simulink model "TST_ECBtn_DD"  (R2016b)
settings: Solver=FixedStepDiscrete  StartTime=0.0  StopTime=simTime  FixedStep=sampleTime  RelTol=1e-3
values from neighbouring files (symbols this model uses):
  testCase = 1    [initTST_ECBtn_DD_001.m]    (also in initTST_ECBtn_DD_002.m = 2)
libraries: simulink x11, UnitTest_Lib x8
settings Model: Creator=xinchangran  LastModifiedBy=xinchangran
settings DebuggingCC: SignalRangeChecking=error
settings ConfigComp: CovEnable=on  RecordCoverage=on  CovFilter=D:\DATA\Control_strategy\build\UnitTest\ECBtn_DD\slcov_output\ECBtn_DD_covfilter.cvf  CovHTMLOptions=-sRT=0  CovHtmlReporting=on  CovSaveCumulativeToWorkspaceVar=on  CovCumulativeVarName=ECBtn_DD_covCumulativeData  CovCumulativeReport=on  CovShowResultsExplorer=off  CovModelRefEnable=on

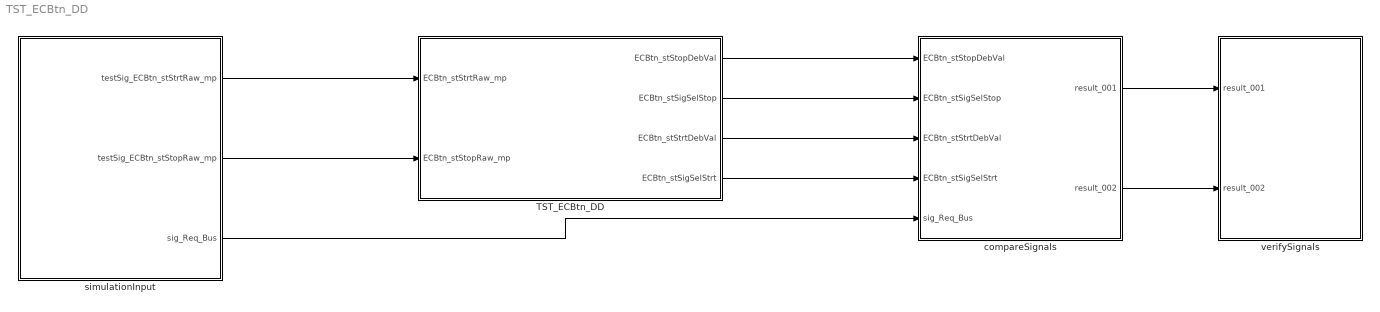
== system TST_ECBtn_DD ==
  TST_ECBtn_DD : Subsystem
  compareSignals : Subsystem
  simulationInput : Subsystem
  verifySignals : Subsystem
  wires:
  simulationInput/1(testSig_ECBtn_stStrtRaw_mp) -> TST_ECBtn_DD/1(ECBtn_stStrtRaw_mp)
  simulationInput/2(testSig_ECBtn_stStopRaw_mp) -> TST_ECBtn_DD/2(ECBtn_stStopRaw_mp)
  TST_ECBtn_DD/1(ECBtn_stStopDebVal) -> compareSignals/1(ECBtn_stStopDebVal)
  TST_ECBtn_DD/2(ECBtn_stSigSelStop) -> compareSignals/2(ECBtn_stSigSelStop)
  TST_ECBtn_DD/3(ECBtn_stStrtDebVal) -> compareSignals/3(ECBtn_stStrtDebVal)
  TST_ECBtn_DD/4(ECBtn_stSigSelStrt) -> compareSignals/4(ECBtn_stSigSelStrt)
  simulationInput/3(sig_Req_Bus) -> compareSignals/5(sig_Req_Bus)
  compareSignals/1(result_001) -> verifySignals/1(result_001)
  compareSignals/2(result_002) -> verifySignals/2(result_002)

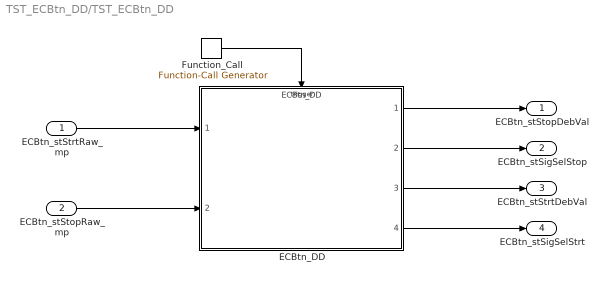
== system TST_ECBtn_DD/TST_ECBtn_DD ==
  ECBtn_stStrtRaw_mp : Inport
  ECBtn_stStopRaw_mp : Inport  Port=2
  ECBtn_DD : ModelReference  ModelNameDialog=ECBtn_DD  SimulationMode=Normal  ModelReferenceVersion=1.74  TriggerPortName=function  TriggerPortTriggerType=function-call  TriggerPortStatesWhenEnabling=held
  Function_Call : simulink/Ports & Subsystems/Function-Call Generator  sample_time=sampleTime  numberOfIterations=1
  ECBtn_stStopDebVal : Outport
  ECBtn_stSigSelStop : Outport  Port=2
  ECBtn_stStrtDebVal : Outport  Port=3
  ECBtn_stSigSelStrt : Outport  Port=4
  wires:
  Function_Call/1 -> ECBtn_DD/Trigger
  ECBtn_stStrtRaw_mp/1 -> ECBtn_DD/1
  ECBtn_stStopRaw_mp/1 -> ECBtn_DD/2
  ECBtn_DD/1 -> ECBtn_stStopDebVal/1
  ECBtn_DD/2 -> ECBtn_stSigSelStop/1
  ECBtn_DD/3 -> ECBtn_stStrtDebVal/1
  ECBtn_DD/4 -> ECBtn_stSigSelStrt/1

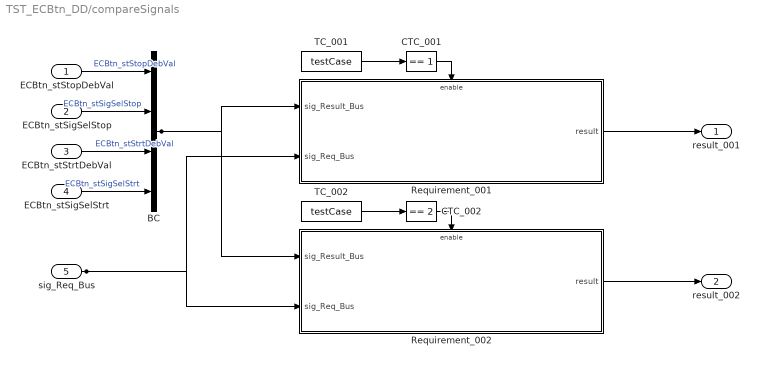
== system TST_ECBtn_DD/compareSignals ==
  ECBtn_stStopDebVal : Inport
  ECBtn_stSigSelStop : Inport  Port=2
  ECBtn_stStrtDebVal : Inport  Port=3
  ECBtn_stSigSelStrt : Inport  Port=4
  sig_Req_Bus : Inport  Port=5
  BC : BusCreator  Inputs=4
  CTC_001 : simulink/Logic and Bit Operations/Compare To Constant  relop===  const=1  OutDataTypeStr=boolean
  CTC_002 : simulink/Logic and Bit Operations/Compare To Constant  relop===  const=2  OutDataTypeStr=boolean
  Requirement_001 : Subsystem
  Requirement_002 : Subsystem
  TC_001 : Constant  Value=testCase
  TC_002 : Constant  Value=testCase
  result_001 : Outport
  result_002 : Outport  Port=2
  wires:
  ECBtn_stStopDebVal/1 -> BC/1  "ECBtn_stStopDebVal"
  ECBtn_stSigSelStop/1 -> BC/2  "ECBtn_stSigSelStop"
  ECBtn_stStrtDebVal/1 -> BC/3  "ECBtn_stStrtDebVal"
  ECBtn_stSigSelStrt/1 -> BC/4  "ECBtn_stSigSelStrt"
  TC_001/1 -> CTC_001/1
  CTC_001/1 -> Requirement_001/Enable
  sig_Req_Bus/1 -> Requirement_001/2(sig_Req_Bus), Requirement_002/2(sig_Req_Bus)
  BC/1 -> Requirement_001/1(sig_Result_Bus), Requirement_002/1(sig_Result_Bus)
  Requirement_001/1(result) -> result_001/1
  TC_002/1 -> CTC_002/1
  CTC_002/1 -> Requirement_002/Enable
  Requirement_002/1(result) -> result_002/1

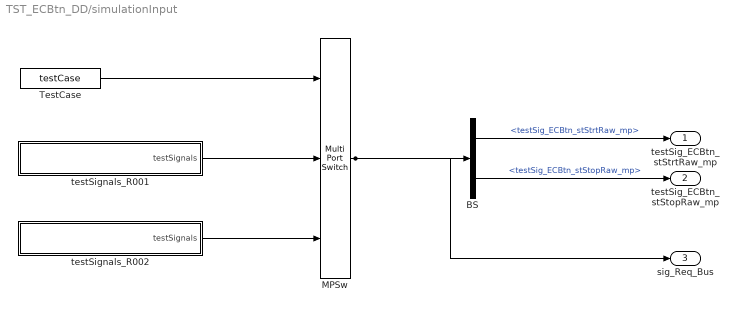
== system TST_ECBtn_DD/simulationInput ==
  BS : BusSelector  OutputSignals=testSig_ECBtn_stStrtRaw_mp,testSig_ECBtn_stStopRaw_mp
  MPSw : MultiPortSwitch  Inputs=2  SaturateOnIntegerOverflow=on  InputSameDT=on
  TestCase : Constant  Value=testCase
  testSignals_R001 : Subsystem
  testSignals_R002 : Subsystem
  testSig_ECBtn_stStrtRaw_mp : Outport
  testSig_ECBtn_stStopRaw_mp : Outport  Port=2
  sig_Req_Bus : Outport  Port=3
  wires:
  BS/1 -> testSig_ECBtn_stStrtRaw_mp/1  "<testSig_ECBtn_stStrtRaw_mp>"
  BS/2 -> testSig_ECBtn_stStopRaw_mp/1  "<testSig_ECBtn_stStopRaw_mp>"
  MPSw/1 -> BS/1, sig_Req_Bus/1
  TestCase/1 -> MPSw/1
  testSignals_R001/1(testSignals) -> MPSw/2
  testSignals_R002/1(testSignals) -> MPSw/3

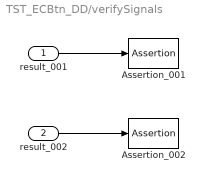
== system TST_ECBtn_DD/verifySignals ==
  result_001 : Inport
  result_002 : Inport  Port=2
  Assertion_001 : Assertion  Enabled=off
  Assertion_002 : Assertion  Enabled=off
  wires:
  result_001/1 -> Assertion_001/1
  result_002/1 -> Assertion_002/1

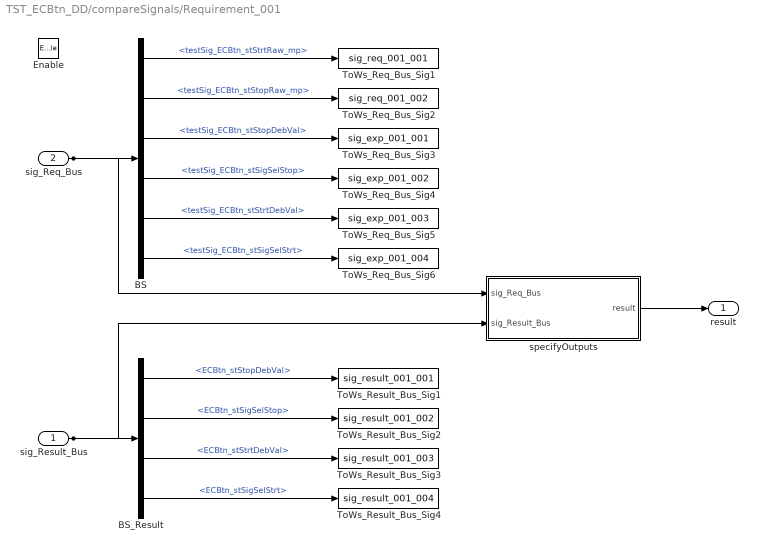
== system TST_ECBtn_DD/compareSignals/Requirement_001 ==
  sig_Result_Bus : Inport
  sig_Req_Bus : Inport  Port=2
  Enable : EnablePort
  BS : BusSelector  OutputSignals=testSig_ECBtn_stStrtRaw_mp,testSig_ECBtn_stStopRaw_mp,testSig_ECBtn_stStopDebVal,testSig_ECBtn_stSigSelStop,testSig_ECBtn_stStrtDebVal,testSig_ECBtn_stSigSelStrt
  BS_Result : BusSelector  OutputSignals=ECBtn_stStopDebVal,ECBtn_stSigSelStop,ECBtn_stStrtDebVal,ECBtn_stSigSelStrt
  ToWs_Req_Bus_Sig1 : ToWorkspace  VariableName=sig_req_001_001  SaveFormat=Structure With Time
  ToWs_Req_Bus_Sig2 : ToWorkspace  VariableName=sig_req_001_002  SaveFormat=Structure With Time
  ToWs_Req_Bus_Sig3 : ToWorkspace  VariableName=sig_exp_001_001  SaveFormat=Structure With Time
  ToWs_Req_Bus_Sig4 : ToWorkspace  VariableName=sig_exp_001_002  SaveFormat=Structure With Time
  ToWs_Req_Bus_Sig5 : ToWorkspace  VariableName=sig_exp_001_003  SaveFormat=Structure With Time
  ToWs_Req_Bus_Sig6 : ToWorkspace  VariableName=sig_exp_001_004  SaveFormat=Structure With Time
  ToWs_Result_Bus_Sig1 : ToWorkspace  VariableName=sig_result_001_001  SaveFormat=Structure With Time
  ToWs_Result_Bus_Sig2 : ToWorkspace  VariableName=sig_result_001_002  SaveFormat=Structure With Time
  ToWs_Result_Bus_Sig3 : ToWorkspace  VariableName=sig_result_001_003  SaveFormat=Structure With Time
  ToWs_Result_Bus_Sig4 : ToWorkspace  VariableName=sig_result_001_004  SaveFormat=Structure With Time
  specifyOutputs : Subsystem
  result : Outport
  wires:
  sig_Req_Bus/1 -> BS/1, specifyOutputs/1(sig_Req_Bus)
  BS/1 -> ToWs_Req_Bus_Sig1/1  "<testSig_ECBtn_stStrtRaw_mp>"
  BS/2 -> ToWs_Req_Bus_Sig2/1  "<testSig_ECBtn_stStopRaw_mp>"
  BS/3 -> ToWs_Req_Bus_Sig3/1  "<testSig_ECBtn_stStopDebVal>"
  BS/4 -> ToWs_Req_Bus_Sig4/1  "<testSig_ECBtn_stSigSelStop>"
  BS/5 -> ToWs_Req_Bus_Sig5/1  "<testSig_ECBtn_stStrtDebVal>"
  BS/6 -> ToWs_Req_Bus_Sig6/1  "<testSig_ECBtn_stSigSelStrt>"
  sig_Result_Bus/1 -> BS_Result/1, specifyOutputs/2(sig_Result_Bus)
  BS_Result/1 -> ToWs_Result_Bus_Sig1/1  "<ECBtn_stStopDebVal>"
  BS_Result/2 -> ToWs_Result_Bus_Sig2/1  "<ECBtn_stSigSelStop>"
  BS_Result/3 -> ToWs_Result_Bus_Sig3/1  "<ECBtn_stStrtDebVal>"
  BS_Result/4 -> ToWs_Result_Bus_Sig4/1  "<ECBtn_stSigSelStrt>"
  specifyOutputs/1(result) -> result/1

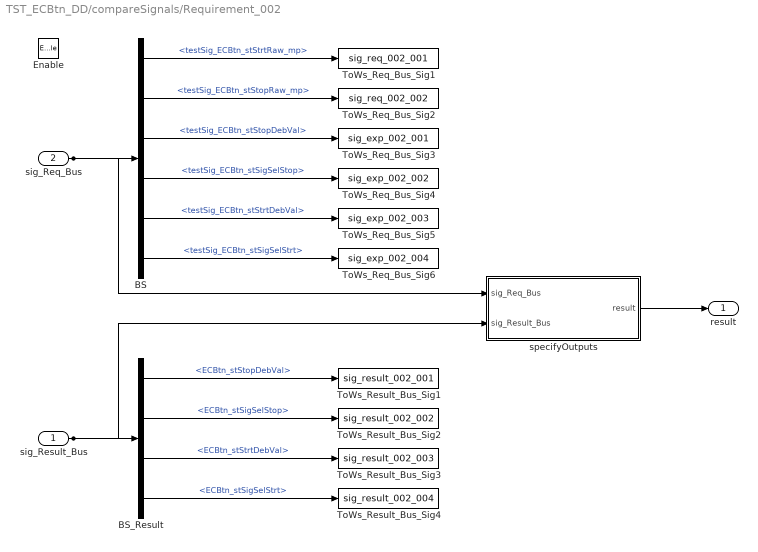
== system TST_ECBtn_DD/compareSignals/Requirement_002 ==
  sig_Result_Bus : Inport
  sig_Req_Bus : Inport  Port=2
  Enable : EnablePort
  BS : BusSelector  OutputSignals=testSig_ECBtn_stStrtRaw_mp,testSig_ECBtn_stStopRaw_mp,testSig_ECBtn_stStopDebVal,testSig_ECBtn_stSigSelStop,testSig_ECBtn_stStrtDebVal,testSig_ECBtn_stSigSelStrt
  BS_Result : BusSelector  OutputSignals=ECBtn_stStopDebVal,ECBtn_stSigSelStop,ECBtn_stStrtDebVal,ECBtn_stSigSelStrt
  ToWs_Req_Bus_Sig1 : ToWorkspace  VariableName=sig_req_002_001  SaveFormat=Structure With Time
  ToWs_Req_Bus_Sig2 : ToWorkspace  VariableName=sig_req_002_002  SaveFormat=Structure With Time
  ToWs_Req_Bus_Sig3 : ToWorkspace  VariableName=sig_exp_002_001  SaveFormat=Structure With Time
  ToWs_Req_Bus_Sig4 : ToWorkspace  VariableName=sig_exp_002_002  SaveFormat=Structure With Time
  ToWs_Req_Bus_Sig5 : ToWorkspace  VariableName=sig_exp_002_003  SaveFormat=Structure With Time
  ToWs_Req_Bus_Sig6 : ToWorkspace  VariableName=sig_exp_002_004  SaveFormat=Structure With Time
  ToWs_Result_Bus_Sig1 : ToWorkspace  VariableName=sig_result_002_001  SaveFormat=Structure With Time
  ToWs_Result_Bus_Sig2 : ToWorkspace  VariableName=sig_result_002_002  SaveFormat=Structure With Time
  ToWs_Result_Bus_Sig3 : ToWorkspace  VariableName=sig_result_002_003  SaveFormat=Structure With Time
  ToWs_Result_Bus_Sig4 : ToWorkspace  VariableName=sig_result_002_004  SaveFormat=Structure With Time
  specifyOutputs : Subsystem
  result : Outport
  wires:
  sig_Req_Bus/1 -> BS/1, specifyOutputs/1(sig_Req_Bus)
  BS/1 -> ToWs_Req_Bus_Sig1/1  "<testSig_ECBtn_stStrtRaw_mp>"
  BS/2 -> ToWs_Req_Bus_Sig2/1  "<testSig_ECBtn_stStopRaw_mp>"
  BS/3 -> ToWs_Req_Bus_Sig3/1  "<testSig_ECBtn_stStopDebVal>"
  BS/4 -> ToWs_Req_Bus_Sig4/1  "<testSig_ECBtn_stSigSelStop>"
  BS/5 -> ToWs_Req_Bus_Sig5/1  "<testSig_ECBtn_stStrtDebVal>"
  BS/6 -> ToWs_Req_Bus_Sig6/1  "<testSig_ECBtn_stSigSelStrt>"
  sig_Result_Bus/1 -> BS_Result/1, specifyOutputs/2(sig_Result_Bus)
  BS_Result/1 -> ToWs_Result_Bus_Sig1/1  "<ECBtn_stStopDebVal>"
  BS_Result/2 -> ToWs_Result_Bus_Sig2/1  "<ECBtn_stSigSelStop>"
  BS_Result/3 -> ToWs_Result_Bus_Sig3/1  "<ECBtn_stStrtDebVal>"
  BS_Result/4 -> ToWs_Result_Bus_Sig4/1  "<ECBtn_stSigSelStrt>"
  specifyOutputs/1(result) -> result/1

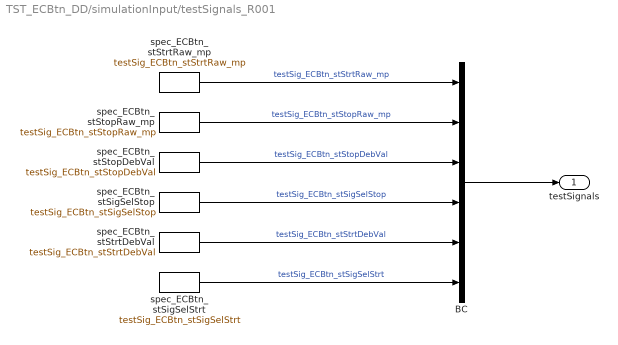
== system TST_ECBtn_DD/simulationInput/testSignals_R001 ==
  BC : BusCreator  Inputs=6
  spec_ECBtn_stSigSelStop : FromWorkspace  VariableName=testSig_ECBtn_stSigSelStop  Interpolate=off  OutputAfterFinalValue=Holding final value
  spec_ECBtn_stSigSelStrt : FromWorkspace  VariableName=testSig_ECBtn_stSigSelStrt  Interpolate=off  OutputAfterFinalValue=Holding final value
  spec_ECBtn_stStopDebVal : FromWorkspace  VariableName=testSig_ECBtn_stStopDebVal  Interpolate=off  OutputAfterFinalValue=Holding final value
  spec_ECBtn_stStopRaw_mp : FromWorkspace  VariableName=testSig_ECBtn_stStopRaw_mp  Interpolate=off  OutputAfterFinalValue=Holding final value
  spec_ECBtn_stStrtDebVal : FromWorkspace  VariableName=testSig_ECBtn_stStrtDebVal  Interpolate=off  OutputAfterFinalValue=Holding final value
  spec_ECBtn_stStrtRaw_mp : FromWorkspace  VariableName=testSig_ECBtn_stStrtRaw_mp  Interpolate=off  OutputAfterFinalValue=Holding final value
  testSignals : Outport
  wires:
  BC/1 -> testSignals/1
  spec_ECBtn_stStrtRaw_mp/1 -> BC/1  "testSig_ECBtn_stStrtRaw_mp"
  spec_ECBtn_stStopRaw_mp/1 -> BC/2  "testSig_ECBtn_stStopRaw_mp"
  spec_ECBtn_stStopDebVal/1 -> BC/3  "testSig_ECBtn_stStopDebVal"
  spec_ECBtn_stSigSelStop/1 -> BC/4  "testSig_ECBtn_stSigSelStop"
  spec_ECBtn_stStrtDebVal/1 -> BC/5  "testSig_ECBtn_stStrtDebVal"
  spec_ECBtn_stSigSelStrt/1 -> BC/6  "testSig_ECBtn_stSigSelStrt"

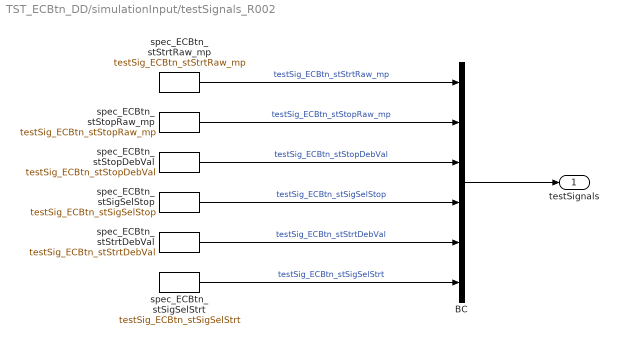
== system TST_ECBtn_DD/simulationInput/testSignals_R002 ==
  BC : BusCreator  Inputs=6
  spec_ECBtn_stSigSelStop : FromWorkspace  VariableName=testSig_ECBtn_stSigSelStop  Interpolate=off  OutputAfterFinalValue=Holding final value
  spec_ECBtn_stSigSelStrt : FromWorkspace  VariableName=testSig_ECBtn_stSigSelStrt  Interpolate=off  OutputAfterFinalValue=Holding final value
  spec_ECBtn_stStopDebVal : FromWorkspace  VariableName=testSig_ECBtn_stStopDebVal  Interpolate=off  OutputAfterFinalValue=Holding final value
  spec_ECBtn_stStopRaw_mp : FromWorkspace  VariableName=testSig_ECBtn_stStopRaw_mp  Interpolate=off  OutputAfterFinalValue=Holding final value
  spec_ECBtn_stStrtDebVal : FromWorkspace  VariableName=testSig_ECBtn_stStrtDebVal  Interpolate=off  OutputAfterFinalValue=Holding final value
  spec_ECBtn_stStrtRaw_mp : FromWorkspace  VariableName=testSig_ECBtn_stStrtRaw_mp  Interpolate=off  OutputAfterFinalValue=Holding final value
  testSignals : Outport
  wires:
  BC/1 -> testSignals/1
  spec_ECBtn_stStrtRaw_mp/1 -> BC/1  "testSig_ECBtn_stStrtRaw_mp"
  spec_ECBtn_stStopRaw_mp/1 -> BC/2  "testSig_ECBtn_stStopRaw_mp"
  spec_ECBtn_stStopDebVal/1 -> BC/3  "testSig_ECBtn_stStopDebVal"
  spec_ECBtn_stSigSelStop/1 -> BC/4  "testSig_ECBtn_stSigSelStop"
  spec_ECBtn_stStrtDebVal/1 -> BC/5  "testSig_ECBtn_stStrtDebVal"
  spec_ECBtn_stSigSelStrt/1 -> BC/6  "testSig_ECBtn_stSigSelStrt"

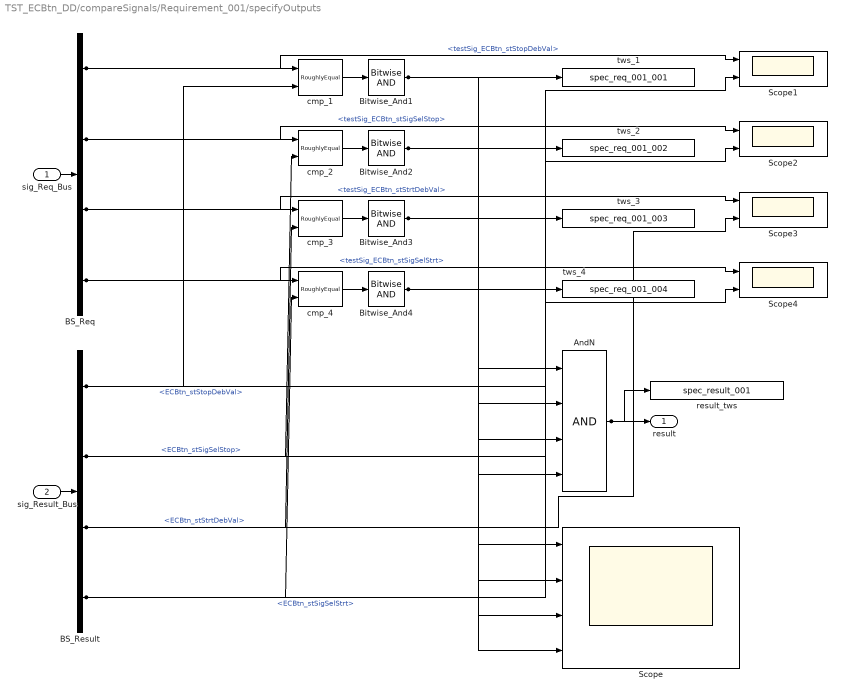
== system TST_ECBtn_DD/compareSignals/Requirement_001/specifyOutputs ==
  sig_Req_Bus : Inport
  sig_Result_Bus : Inport  Port=2
  AndN : Logic  Inputs=4
  BS_Req : BusSelector  OutputSignals=testSig_ECBtn_stStopDebVal,testSig_ECBtn_stSigSelStop,testSig_ECBtn_stStrtDebVal,testSig_ECBtn_stSigSelStrt
  BS_Result : BusSelector  OutputSignals=ECBtn_stStopDebVal,ECBtn_stSigSelStop,ECBtn_stStrtDebVal,ECBtn_stSigSelStrt
  Bitwise_And{1..4} (4 alike) : simulink/Logic and Bit Operations/Bitwise Operator  logicop=AND  UseBitMask=off  BitMask=bin2dec('11011001')  BitMaskRealWorld=Stored Integer
  Scope : Scope  NumInputPorts=4
  Scope{1..4} (4 alike) : Scope  NumInputPorts=2
  cmp_{1..4} (4 alike) : UnitTest_Lib/RoughlyEqual  slope=0.1
  result_tws : ToWorkspace  VariableName=spec_result_001
  tws_1 : ToWorkspace  VariableName=spec_req_001_001
  tws_2 : ToWorkspace  VariableName=spec_req_001_002
  tws_3 : ToWorkspace  VariableName=spec_req_001_003
  tws_4 : ToWorkspace  VariableName=spec_req_001_004
  result : Outport
  wires:
  sig_Req_Bus/1 -> BS_Req/1
  sig_Result_Bus/1 -> BS_Result/1
  AndN/1 -> result/1, result_tws/1
  BS_Req/1 -> cmp_1/1, Scope1/1  "<testSig_ECBtn_stStopDebVal>"
  BS_Result/1 -> cmp_1/2, Scope1/2  "<ECBtn_stStopDebVal>"
  cmp_1/1 -> Bitwise_And1/1
  Bitwise_And1/1 -> tws_1/1, AndN/1, Scope/1
  BS_Req/2 -> cmp_2/1, Scope2/1  "<testSig_ECBtn_stSigSelStop>"
  BS_Result/2 -> cmp_2/2, Scope2/2  "<ECBtn_stSigSelStop>"
  cmp_2/1 -> Bitwise_And2/1
  Bitwise_And2/1 -> tws_2/1, AndN/2, Scope/2
  BS_Req/3 -> cmp_3/1, Scope3/1  "<testSig_ECBtn_stStrtDebVal>"
  BS_Result/3 -> cmp_3/2, Scope3/2  "<ECBtn_stStrtDebVal>"
  cmp_3/1 -> Bitwise_And3/1
  Bitwise_And3/1 -> tws_3/1, AndN/3, Scope/3
  BS_Req/4 -> cmp_4/1, Scope4/1  "<testSig_ECBtn_stSigSelStrt>"
  BS_Result/4 -> cmp_4/2, Scope4/2  "<ECBtn_stSigSelStrt>"
  cmp_4/1 -> Bitwise_And4/1
  Bitwise_And4/1 -> tws_4/1, AndN/4, Scope/4

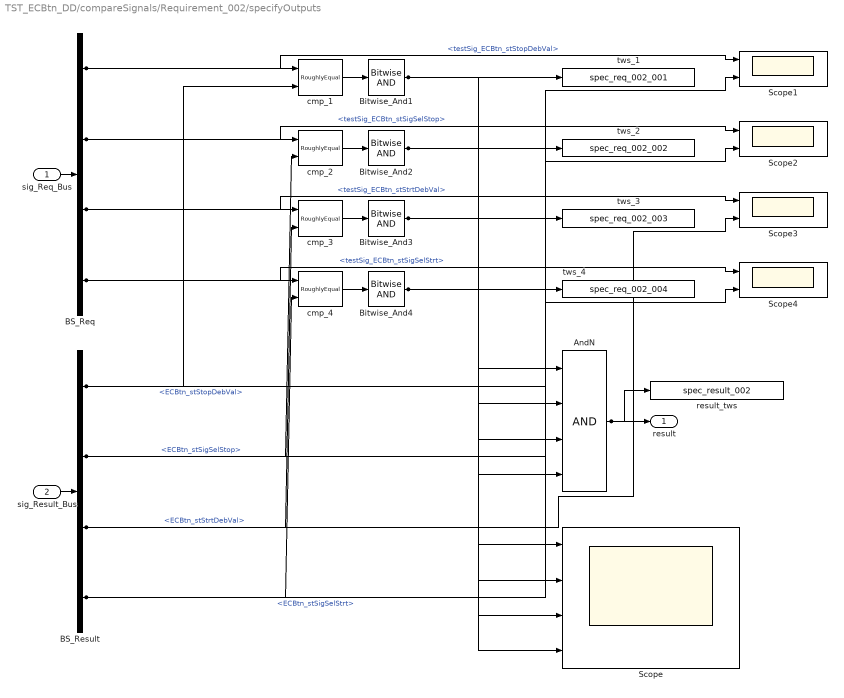
== system TST_ECBtn_DD/compareSignals/Requirement_002/specifyOutputs ==
  sig_Req_Bus : Inport
  sig_Result_Bus : Inport  Port=2
  AndN : Logic  Inputs=4
  BS_Req : BusSelector  OutputSignals=testSig_ECBtn_stStopDebVal,testSig_ECBtn_stSigSelStop,testSig_ECBtn_stStrtDebVal,testSig_ECBtn_stSigSelStrt
  BS_Result : BusSelector  OutputSignals=ECBtn_stStopDebVal,ECBtn_stSigSelStop,ECBtn_stStrtDebVal,ECBtn_stSigSelStrt
  Bitwise_And{1..4} (4 alike) : simulink/Logic and Bit Operations/Bitwise Operator  logicop=AND  UseBitMask=off  BitMask=bin2dec('11011001')  BitMaskRealWorld=Stored Integer
  Scope : Scope  NumInputPorts=4
  Scope{1..4} (4 alike) : Scope  NumInputPorts=2
  cmp_{1..4} (4 alike) : UnitTest_Lib/RoughlyEqual  slope=0.1
  result_tws : ToWorkspace  VariableName=spec_result_002
  tws_1 : ToWorkspace  VariableName=spec_req_002_001
  tws_2 : ToWorkspace  VariableName=spec_req_002_002
  tws_3 : ToWorkspace  VariableName=spec_req_002_003
  tws_4 : ToWorkspace  VariableName=spec_req_002_004
  result : Outport
  wires:
  sig_Req_Bus/1 -> BS_Req/1
  sig_Result_Bus/1 -> BS_Result/1
  AndN/1 -> result/1, result_tws/1
  BS_Req/1 -> cmp_1/1, Scope1/1  "<testSig_ECBtn_stStopDebVal>"
  BS_Result/1 -> cmp_1/2, Scope1/2  "<ECBtn_stStopDebVal>"
  cmp_1/1 -> Bitwise_And1/1
  Bitwise_And1/1 -> tws_1/1, AndN/1, Scope/1
  BS_Req/2 -> cmp_2/1, Scope2/1  "<testSig_ECBtn_stSigSelStop>"
  BS_Result/2 -> cmp_2/2, Scope2/2  "<ECBtn_stSigSelStop>"
  cmp_2/1 -> Bitwise_And2/1
  Bitwise_And2/1 -> tws_2/1, AndN/2, Scope/2
  BS_Req/3 -> cmp_3/1, Scope3/1  "<testSig_ECBtn_stStrtDebVal>"
  BS_Result/3 -> cmp_3/2, Scope3/2  "<ECBtn_stStrtDebVal>"
  cmp_3/1 -> Bitwise_And3/1
  Bitwise_And3/1 -> tws_3/1, AndN/3, Scope/3
  BS_Req/4 -> cmp_4/1, Scope4/1  "<testSig_ECBtn_stSigSelStrt>"
  BS_Result/4 -> cmp_4/2, Scope4/2  "<ECBtn_stSigSelStrt>"
  cmp_4/1 -> Bitwise_And4/1
  Bitwise_And4/1 -> tws_4/1, AndN/4, Scope/4
